simulink model "Full_Wave_Rectifier_FullController_RLoad2015"  (R2015a)
settings: Solver=ode45  SolverMode=SingleTasking  StartTime=0.0  StopTime=0.06  MaxStep=1e-4  RelTol=1e-3
libraries: powerlib x13
settings Model: CovMetricSettings=dwe  CovHtmlReporting=off  covSaveCumulativeToWorkspaceVar=off  CovSaveSingleToWorkspaceVar=off  CovExternalEMLEnable=on  Creator=sepykian  LastModifiedBy=A.hey
settings DataIOCC: LimitDataPoints=off  SaveFormat=Dataset
settings DebuggingCC: SFUnexpectedBacktrackingDiag=error  SFNoUnconditionalDefaultTransitionDiag=error
settings HardwareCC: ProdBitPerPointer=64  ProdLargestAtomicFloat=Float  ProdIntDivRoundTo=Zero  ProdEndianess=LittleEndian  ProdHWDeviceType=Specified
settings ModelReferenceCC: PropagateSignalLabelsOutOfModel=on
settings GRTTargetCC: TargetLangStandard=C99 (ISO)  GeneratePreprocessorConditionals=Use local settings
settings ConfigurationSet: Description=Simscape Multibody

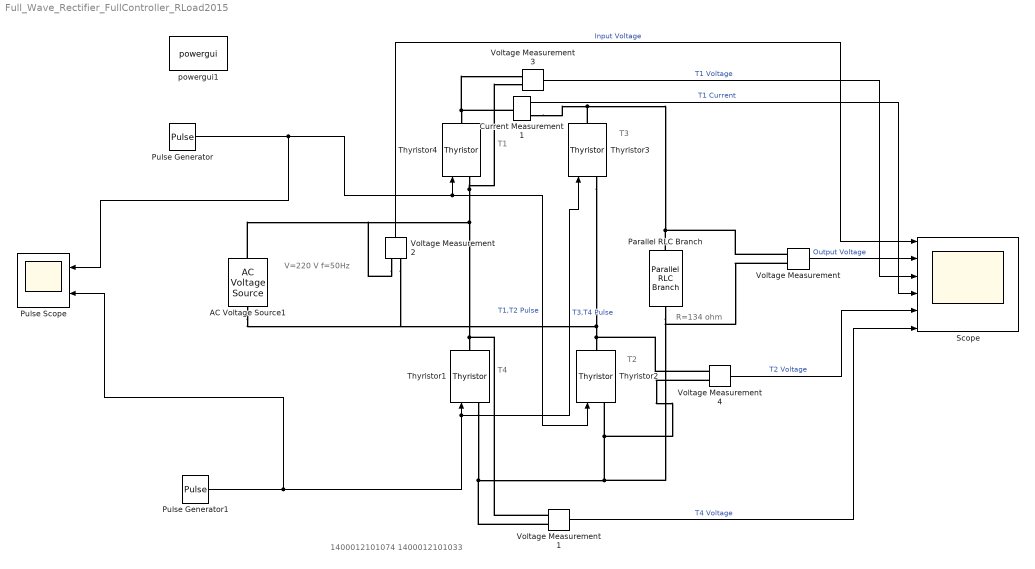
== system Full_Wave_Rectifier_FullController_RLoad2015 ==
  note: R=134 ohm
  note: 1400012101074
      | 1400012101033
  note: V=220 V
      | f=50Hz
  note: T3
  note: T1
  note: T2
  note: T4
  AC Voltage Source1 : powerlib/Electrical Sources/AC Voltage Source  Amplitude=220  Phase=0  Frequency=50  SampleTime=0  Measurements=None  BusType=swing  Pref=10e3  Qref=0  Qmin=-inf  Qmax=+inf
  Current Measurement1 : powerlib/Measurements/Current Measurement  PhasorSimulation=off  OutputType=Complex  PSBequivalent=0
  Parallel RLC Branch : powerlib/Elements/Parallel RLC Branch  LConnTagsString=a  RConnTagsString=__new0  BranchType=R  Resistance=134  Inductance=1e-3  SetiL0=off  InitialCurrent=0  Capacitance=1e-6  Setx0=off  InitialVoltage=0  Measurements=None
  Pulse Generator : DiscretePulseGenerator  PulseType=Time based  Amplitude=10  Period=0.02  PulseWidth=25  PhaseDelay=0.005
  Pulse Generator1 : DiscretePulseGenerator  PulseType=Time based  Amplitude=10  Period=0.02  PulseWidth=25  PhaseDelay=0.015
  Pulse Scope : Scope  NumInputPorts=2
      settings: TimeRange=auto  ShowLegends=on  MaxDataPoints=5000  SaveToWorkspace=off  YMin=-1.25~-1.25  YMax=11.25~11.25  SampleTime=-1
  "Scope " : Scope  NumInputPorts=6
      settings: TimeRange=auto  ShowLegends=on  MaxDataPoints=5000  SaveToWorkspace=off  SaveName=ScopeData2  YMin=-275.00000~-27.47448~-261.13516~-0.4802~-261.13516~-261.13516  YMax=275.00000~247.27032~151.23724~2.12047~151.23724~151.23724  SampleTime=-1
  Thyristor{1..4} (4 alike) : powerlib/Power Electronics/Thyristor  Ron=0.001  Lon=0  Vf=0.1  IC=0  Rs=500  Cs=250e-9  Measurements=off
  Voltage Measurement{,1..4} (5 alike) : powerlib/Measurements/Voltage Measurement  PhasorSimulation=off  OutputType=Complex  PSBequivalent=0
  powergui1 : powerlib/powergui  Priority=1  SimulationMode=Continuous  SampleTime=50e-6  frequency=60  Iterations=50  frequencyindice=50  Pbase=100e6  ErrMax=1e-4  UnitsV=kV  UnitsW=MW  buscounter=0  FunctionMessages=off  echomessages=off  EnableUseOfTLC=off  CurrentSourceSwitches=off  DisableSnubberDevices=off  DisableRonSwitches=off  DisableVfSwitches=off  DisplayEquations=off  SolverType=Tustin/Backward Euler (TBE)  Interpol=off  ExternalGateDelay=off  methode=off  Ts=100  x0status=blocks  SPID=on  SwTol=0  HookPort=off  RestoreLinks=warning  ResistiveCurrentMeasurement=off  Frange=[0:2:500]  Ylog=off  Xlog=on  ShowGrid=off  save=off  variable=ZData  structure=0  ZoomFFT=off  StartTime=0.0  cycles=1  DisplayStyle=1  fundamental=60  FreqAxis=off  MaxFrequency=1000  frequencyindicesteady=1  RmsSteady=1  display=off
  wires:
  Pulse Generator/1 -> Pulse Scope/1, Thyristor2/1, Thyristor4/1  "T1,T2 Pulse"
  Pulse Generator1/1 -> Pulse Scope/2, Thyristor3/1, Thyristor1/1  "T3,T4 Pulse"
  Voltage Measurement2/1 -> "Scope "/1  "Input Voltage"
  Voltage Measurement/1 -> "Scope "/2  "Output Voltage"
  Voltage Measurement3/1 -> "Scope "/3  "T1 Voltage"
  Current Measurement1/1 -> "Scope "/4  "T1 Current"
  Voltage Measurement4/1 -> "Scope "/5  "T2 Voltage"
  Voltage Measurement1/1 -> "Scope "/6  "T4 Voltage"
  connections:
  Thyristor4/LConn1 -- Voltage Measurement3/LConn1 -- AC Voltage Source1/RConn1 -- Voltage Measurement2/LConn1 -- Voltage Measurement1/LConn2 -- Thyristor1/RConn1
  Thyristor3/LConn1 -- Voltage Measurement2/LConn2 -- AC Voltage Source1/LConn1 -- Voltage Measurement4/LConn2 -- Thyristor2/RConn1
  Thyristor3/RConn1 -- Parallel RLC Branch/LConn1 -- Voltage Measurement/LConn1 -- Current Measurement1/RConn1
  Thyristor1/LConn1 -- Voltage Measurement1/LConn1 -- Parallel RLC Branch/RConn1 -- Voltage Measurement/LConn2 -- Voltage Measurement4/LConn1 -- Thyristor2/LConn1
  Thyristor4/RConn1 -- Voltage Measurement3/LConn2 -- Current Measurement1/LConn1
